simulink model "PID_joint1"  (R2017b)
settings: Solver=ode4  StartTime=0.0  StopTime=0.42289  FixedStep=0.001  RelTol=1e-3
settings Model: Creator=84935  LastModifiedBy=84935

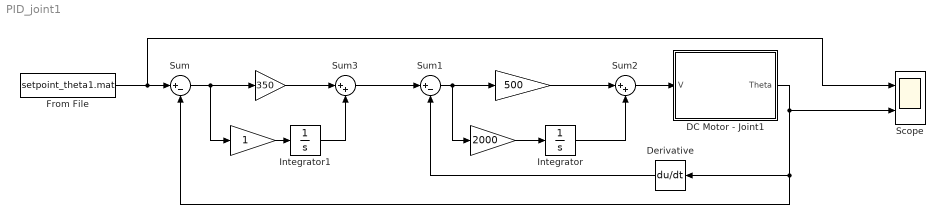
== system PID_joint1 ==
  " " : Gain  Gain=350
  " " : Gain
  " " : Gain  Gain=2000
  " " : Gain  Gain=500
  DC Motor - Joint1 : Subsystem  mask{L=0.012342, R=3.2645, Ki=1.1895, Jeff=0.01829, Beff=0.019, Kb=1.1895, N=200}
  Derivative : Derivative
  From File : FromFile  FileName=setpoint_theta1.mat  SampleTime=0
  Integrator : Integrator
  Integrator1 : Integrator
  Scope : Scope  NumInputPorts=2
  Sum : Sum  Inputs=|+-
  Sum1 : Sum  Inputs=|+-
  Sum2 : Sum  Inputs=|++
  Sum3 : Sum  Inputs=|++
  wires:
  " "/1 -> Sum3/1
  Sum/1 -> " "/1, " "/1
  Integrator1/1 -> Sum3/2
  " "/1 -> Integrator1/1
  From File/1 -> Scope/1, Sum/1
  Integrator/1 -> Sum2/2
  " "/1 -> Sum2/1
  Derivative/1 -> Sum1/2
  " "/1 -> Integrator/1
  Sum1/1 -> " "/1, " "/1
  DC Motor - Joint1/1(Theta) -> Scope/2, Sum/2, Derivative/1
  Sum3/1 -> Sum1/1
  Sum2/1 -> DC Motor - Joint1/1(V)

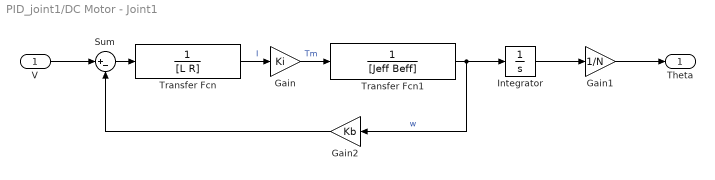
== system PID_joint1/DC Motor - Joint1 ==
  V : Inport
  Gain : Gain  Gain=Ki
  Gain1 : Gain  Gain=1/N
  Gain2 : Gain  Gain=Kb
  Integrator : Integrator
  Sum : Sum  Inputs=|+-
  Transfer Fcn : TransferFcn  Denominator=[L R]
  Transfer Fcn1 : TransferFcn  Denominator=[Jeff Beff]
  Theta : Outport
  wires:
  Integrator/1 -> Gain1/1
  Transfer Fcn1/1 -> Integrator/1, Gain2/1  "w"
  V/1 -> Sum/1
  Gain2/1 -> Sum/2
  Gain/1 -> Transfer Fcn1/1  "Tm"
  Gain1/1 -> Theta/1
  Sum/1 -> Transfer Fcn/1
  Transfer Fcn/1 -> Gain/1  "I"
